simulink model "T2_unstable_gain"  (R2025a)
settings: Solver=VariableStepAuto  StartTime=0.0  StopTime=100  RelTol=1e-3
undefined symbols (not defined in the file): Gm
settings Model: Creator=abhi  LastModifiedBy=abhi

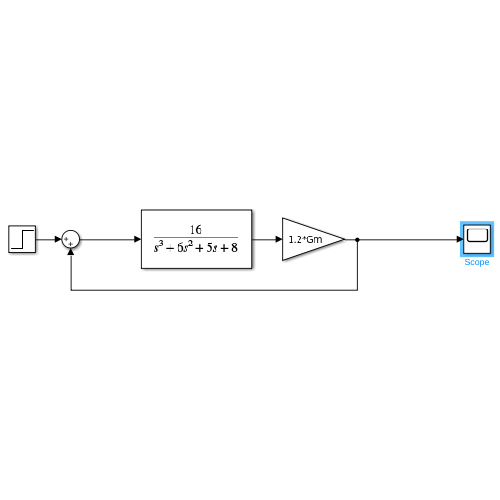
[thumbnail: Simulink's stored preview of the top-level diagram]
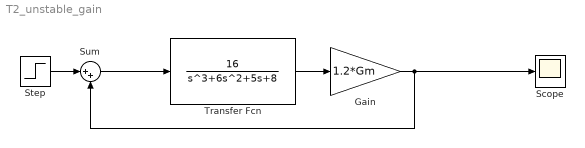
== system T2_unstable_gain ==
  Gain : Gain  Gain=1.2*Gm
  Scope : Scope
      settings: ActiveDisplayYMinimum=-1.4591834013112355E+54  ActiveDisplayYMaximum=1.3132650611801123E+55
  Step : Step  SampleTime=0
  Sum : Sum  Inputs=|++
  Transfer Fcn : TransferFcn  Numerator=[16]  Denominator=[1 6 5 8]
  wires:
  Transfer Fcn/1 -> Gain/1
  Sum/1 -> Transfer Fcn/1
  Step/1 -> Sum/1
  Gain/1 -> Sum/2, Scope/1
